simulink model "R2023b_Sim_Knickarmroboter_AndreasPaul"  (R2023b)
settings: Solver=ode45  StartTime=0.0  StopTime=2  MaxStep=3e-3  RelTol=1e-4  AbsTol=1e-7
values from neighbouring files (symbols this model uses):
  D = [1,0 ... (first row only)    [Initialisierung_Kickarmroboter.m]
  F_s1 = 8.5e-4    (= 0.00085)    [Initialisierung_Kickarmroboter.m]
  F_s2 = 3.2e-4    (= 0.00032)    [Initialisierung_Kickarmroboter.m]
  g = 9.81    [Initialisierung_Kickarmroboter.m]
  I = [1,0 ... (first row only)    [Initialisierung_Kickarmroboter.m]
  I1 = 0.0309    [Initialisierung_Kickarmroboter.m]
  I2 = 0.0045    [Initialisierung_Kickarmroboter.m]
  l1 = 0.16    [Initialisierung_Kickarmroboter.m]
  l2 = 0.128    [Initialisierung_Kickarmroboter.m]
  m1 = 0.1817    [Initialisierung_Kickarmroboter.m]
  m2 = 0.0944    [Initialisierung_Kickarmroboter.m]
  mu_v1 = 3.843e-6    (= 3.843e-06)    [Initialisierung_Kickarmroboter.m]
  mu_v2 = 3.887e-6    (= 3.887e-06)    [Initialisierung_Kickarmroboter.m]
  P = [1,0 ... (first row only)    [Initialisierung_Kickarmroboter.m]
  tau_delta_alpha = 0.1    [Initialisierung_Kickarmroboter.m]
  tau_delta_beta = 0.1    [Initialisierung_Kickarmroboter.m]
  x0 = [-2.5658; 0.2465; 0; 0]    [Initialisierung_Kickarmroboter.m]
libraries: simulink x1
settings Model: Creator=apaul  LastModifiedBy=apaul
settings RTWCC: GPUComputeCapability=5.0

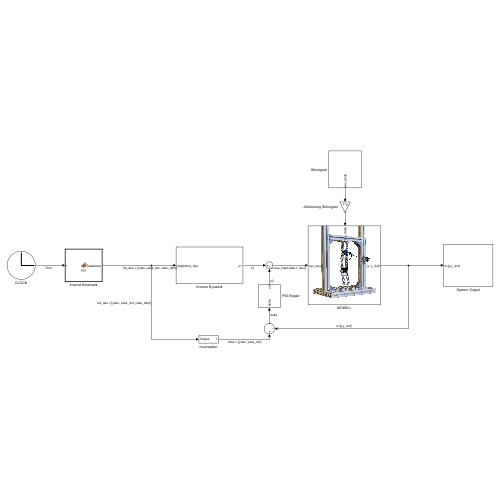
[thumbnail: Simulink's stored preview of the top-level diagram]
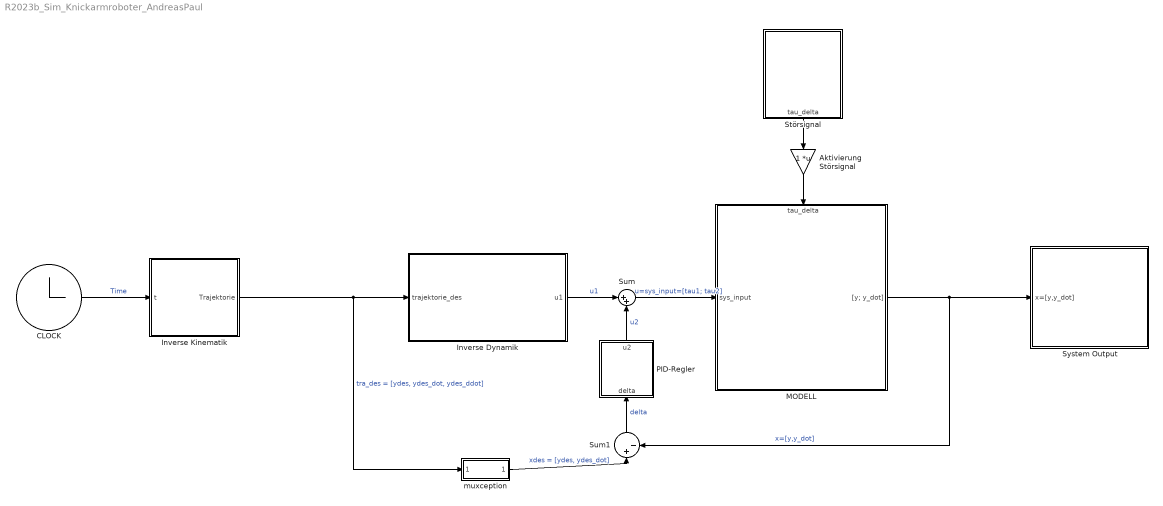
== system R2023b_Sim_Knickarmroboter_AndreasPaul ==
  Aktivierung Störsignal : Gain  Multiplication=Matrix(K*u)
  CLOCK : Clock
  Inverse Dynamik : Subsystem
  Inverse Kinematik : MATLAB Function  TreatAsAtomicUnit=on
  MODELL : Subsystem
      settings: PortSchema="{\"entries\":[{\"content\":{\"sides\":[{\"content\":{\"connectorIds\":[\"In1\"]},\"type\":\"ConnectorPlacement.EquallySpacedRectSide\",\"uuid\":\"e44e4c36-5739-4e55-a6ec-ca88d6f73c34\"},{\"content\":{\"connectorIds\":[\"Out1\"],\"side\":\"RIGHT\"},\"type\":\"ConnectorPlacement.EquallySpacedRectSide\",\"uuid\":\"5e6c41ef-5797-46fa-899e-46ee2542736a\"},{\"content\":{\"connectorIds\":[\"In2\"],\"side\":\"TOP\"},\"type\":\"ConnectorPlacement.EquallySpacedRectSide\",\"uuid\":\"f6ef0a2a-5723-4456-9106-f5bf4cdb5031\"}]},\"type\":\"ConnectorPlacement.EquallySpacedConnector\",\"uuid\":\"21cb76c5-3abe-4316-bc4d-4651aaedd4ba\"}],\"packageUris\":[\"http://schema.mathworks.com/mf0/Connector/R2020b\"],\"version\":\"1.0\"}"
      mask Display: image('Versuchsaufbau.png');
  PID-Regler : Subsystem
  Störsignal : Subsystem
  Sum : Sum  Inputs=|++
  Sum1 : Sum  Inputs=|+-
  System Output : Subsystem
  muxception : Subsystem
  wires:
  Sum/1 -> MODELL/1(sys_input)  "u=sys_input=[tau1; tau2]"
  Sum1/1 -> PID-Regler/1(delta)  "delta"
  MODELL/1("[y; y_dot]") -> System Output/1(x=[y,y_dot]), Sum1/2  "x=[y,y_dot]"
  Inverse Kinematik/1(Trajektorie) -> muxception/1(Output), Inverse Dynamik/1(trajektorie_des)  "tra_des = [ydes, ydes_dot, ydes_ddot]"
  Inverse Dynamik/1(u1) -> Sum/1  "u1"
  muxception/1(Out1) -> Sum1/1  "xdes = [ydes, ydes_dot]"
  CLOCK/1 -> Inverse Kinematik/1(t)  "Time"
  Störsignal/1(tau_delta) -> Aktivierung Störsignal/1
  Aktivierung Störsignal/1 -> MODELL/2(tau_delta)
  PID-Regler/1(u2) -> Sum/2  "u2"

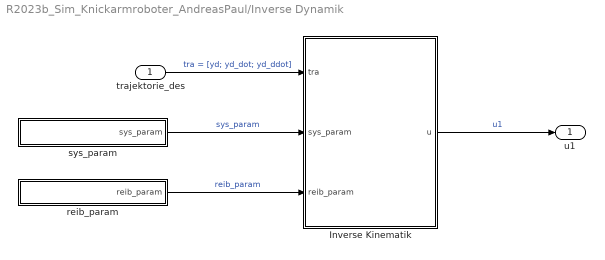
== system R2023b_Sim_Knickarmroboter_AndreasPaul/Inverse Dynamik ==
  trajektorie_des : Inport
  Inverse Kinematik : MATLAB Function  TreatAsAtomicUnit=on
  reib_param : Subsystem
  sys_param : Subsystem
  u1 : Outport
  wires:
  trajektorie_des/1 -> Inverse Kinematik/1(tra)  "tra = [yd; yd_dot; yd_ddot]"
  Inverse Kinematik/1(u) -> u1/1  "u1"
  sys_param/1(sys_param) -> Inverse Kinematik/2(sys_param)  "sys_param"
  reib_param/1(reib_param) -> Inverse Kinematik/3(reib_param)  "reib_param"

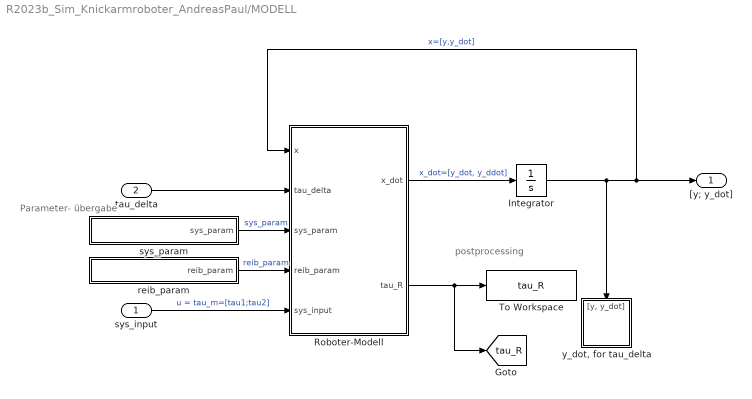
== system R2023b_Sim_Knickarmroboter_AndreasPaul/MODELL ==
  note: postprocessing
  note: Parameter-
      | übergabe
  sys_input : Inport
  tau_delta : Inport  Port=2
  Integrator : Integrator  InitialCondition=x0
  Roboter-Modell : MATLAB Function  TreatAsAtomicUnit=on
  To Workspace : ToWorkspace  VariableName=tau_R  SaveFormat=Timeseries  SampleTime=-1
  reib_param : Subsystem
  sys_param : Subsystem
  "y_dot, for tau_delta" : Subsystem
  "[y; y_dot]" : Outport
  tag scope: tau_R=global
  wires:
  Roboter-Modell/1(x_dot) -> Integrator/1  "x_dot=[y_dot, y_ddot]"
  Integrator/1 -> Roboter-Modell/1(x), "[y; y_dot]"/1, "y_dot, for tau_delta"/1("[y, y_dot]")  "x=[y,y_dot]"
  sys_input/1 -> Roboter-Modell/5(sys_input)  "u = tau_m=[tau1;tau2]"
  sys_param/1(sys_param) -> Roboter-Modell/3(sys_param)  "sys_param"
  reib_param/1(reib_param) -> Roboter-Modell/4(reib_param)  "reib_param"
  tau_delta/1 -> Roboter-Modell/2(tau_delta)
  Roboter-Modell/2(tau_R) -> [tau_R], To Workspace/1

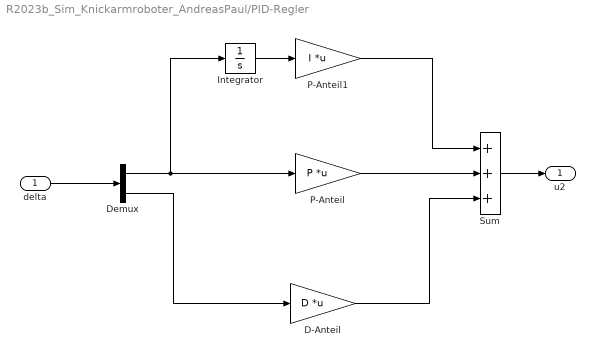
== system R2023b_Sim_Knickarmroboter_AndreasPaul/PID-Regler ==
  delta : Inport
  D-Anteil : Gain  Gain=D  Multiplication=Matrix(K*u)
  Demux : Demux  Outputs=2
  Integrator : Integrator
  P-Anteil : Gain  Gain=P  Multiplication=Matrix(K*u)
  P-Anteil1 : Gain  Gain=I  Multiplication=Matrix(K*u)
  Sum : Sum  Inputs=+++
  u2 : Outport
  wires:
  delta/1 -> Demux/1
  Demux/1 -> P-Anteil/1, Integrator/1
  Demux/2 -> D-Anteil/1
  Integrator/1 -> P-Anteil1/1
  Sum/1 -> u2/1
  P-Anteil1/1 -> Sum/1
  P-Anteil/1 -> Sum/2
  D-Anteil/1 -> Sum/3

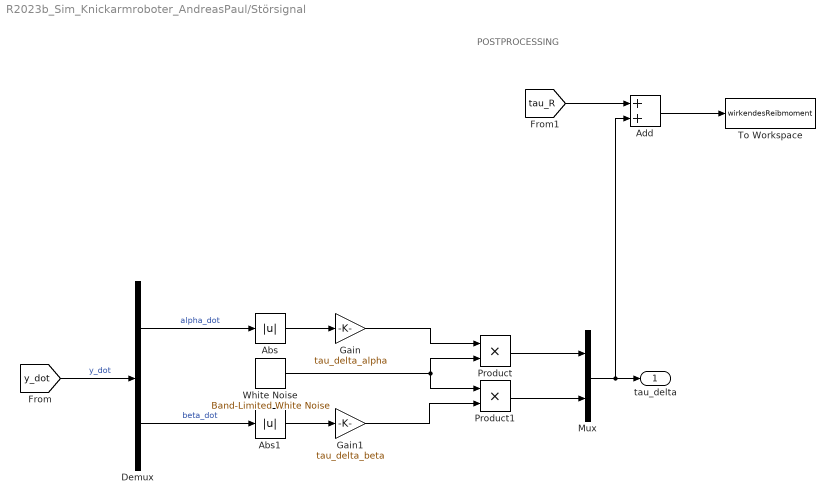
== system R2023b_Sim_Knickarmroboter_AndreasPaul/Störsignal ==
  note: POSTPROCESSING
  Abs : Abs  SaturateOnIntegerOverflow=off
  Abs1 : Abs  SaturateOnIntegerOverflow=off
  Add : Sum
  Demux : Demux  Outputs=2
  Gain : Gain  Gain=tau_delta_alpha
  Gain1 : Gain  Gain=tau_delta_beta
  Mux : Mux  Inputs=2
  Product : Product
  Product1 : Product
  To Workspace : ToWorkspace  VariableName=wirkendesReibmoment  SaveFormat=Timeseries  SampleTime=-1
  White Noise : simulink/Sources/Band-Limited White Noise  Cov=[0.1]  Ts=0.02  seed=[23341]
  tau_delta : Outport
  wires:
  [y_dot] -> Demux/1  "y_dot"
  Demux/1 -> Abs/1  "alpha_dot"
  Demux/2 -> Abs1/1  "beta_dot"
  Abs/1 -> Gain/1
  White Noise/1 -> Product1/1, Product/2
  Abs1/1 -> Gain1/1
  Product1/1 -> Mux/2
  Product/1 -> Mux/1
  Mux/1 -> tau_delta/1, Add/2
  Gain/1 -> Product/1
  Gain1/1 -> Product1/2
  [tau_R] -> Add/1
  Add/1 -> To Workspace/1

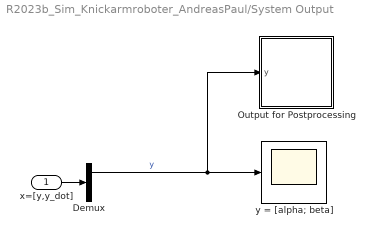
== system R2023b_Sim_Knickarmroboter_AndreasPaul/System Output ==
  x=[y,y_dot] : Inport
  Demux : Demux  Outputs=2
  Output for Postprocessing : Subsystem
  y = [alpha; beta] : Scope
  wires:
  Demux/1 -> Output for Postprocessing/1(y), y = [alpha; beta]/1  "y"
  x=[y,y_dot]/1 -> Demux/1

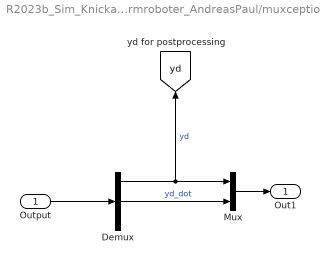
== system R2023b_Sim_Knickarmroboter_AndreasPaul/muxception ==
  Output : Inport
  Demux : Demux  Outputs=3
  Mux : Mux  Inputs=2
  Out1 : Outport
  tag scope: yd=global
  wires:
  Output/1 -> Demux/1
  Demux/1 -> Mux/1, [yd]  "yd"
  Demux/2 -> Mux/2  "yd_dot"
  Mux/1 -> Out1/1

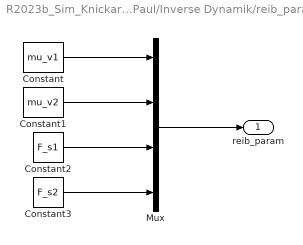
== system R2023b_Sim_Knickarmroboter_AndreasPaul/Inverse Dynamik/reib_param ==
  Constant : Constant  Value=mu_v1
  Constant1 : Constant  Value=mu_v2
  Constant2 : Constant  Value=F_s1
  Constant3 : Constant  Value=F_s2
  Mux : Mux
  reib_param : Outport
  wires:
  Constant3/1 -> Mux/4
  Constant2/1 -> Mux/3
  Constant1/1 -> Mux/2
  Constant/1 -> Mux/1
  Mux/1 -> reib_param/1

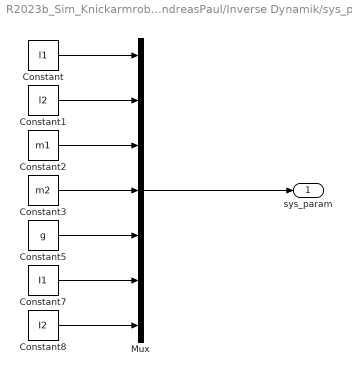
== system R2023b_Sim_Knickarmroboter_AndreasPaul/Inverse Dynamik/sys_param ==
  Constant : Constant  Value=l1
  Constant1 : Constant  Value=l2
  Constant2 : Constant  Value=m1
  Constant3 : Constant  Value=m2
  Constant5 : Constant  Value=g
  Constant7 : Constant  Value=I1
  Constant8 : Constant  Value=I2
  Mux : Mux  Inputs=7
  sys_param : Outport
  wires:
  Constant8/1 -> Mux/7
  Constant7/1 -> Mux/6
  Constant3/1 -> Mux/4
  Constant2/1 -> Mux/3
  Constant1/1 -> Mux/2
  Constant/1 -> Mux/1
  Mux/1 -> sys_param/1
  Constant5/1 -> Mux/5

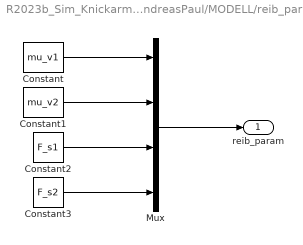
== system R2023b_Sim_Knickarmroboter_AndreasPaul/MODELL/reib_param ==
  Constant : Constant  Value=mu_v1
  Constant1 : Constant  Value=mu_v2
  Constant2 : Constant  Value=F_s1
  Constant3 : Constant  Value=F_s2
  Mux : Mux
  reib_param : Outport
  wires:
  Constant3/1 -> Mux/4
  Constant2/1 -> Mux/3
  Constant1/1 -> Mux/2
  Constant/1 -> Mux/1
  Mux/1 -> reib_param/1

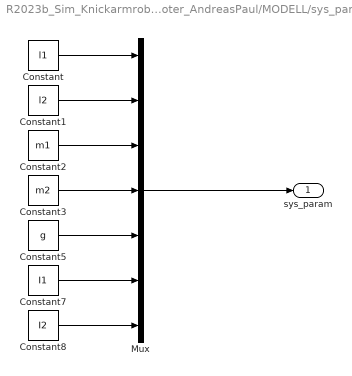
== system R2023b_Sim_Knickarmroboter_AndreasPaul/MODELL/sys_param ==
  Constant : Constant  Value=l1
  Constant1 : Constant  Value=l2
  Constant2 : Constant  Value=m1
  Constant3 : Constant  Value=m2
  Constant5 : Constant  Value=g
  Constant7 : Constant  Value=I1
  Constant8 : Constant  Value=I2
  Mux : Mux  Inputs=7
  sys_param : Outport
  wires:
  Constant8/1 -> Mux/7
  Constant7/1 -> Mux/6
  Constant3/1 -> Mux/4
  Constant2/1 -> Mux/3
  Constant1/1 -> Mux/2
  Constant/1 -> Mux/1
  Mux/1 -> sys_param/1
  Constant5/1 -> Mux/5

== system R2023b_Sim_Knickarmroboter_AndreasPaul/MODELL/y_dot, for tau_delta ==
  "[y, y_dot]" : Inport
  Demux : Demux  Outputs=2
  tag scope: y_dot=global
  wires:
  "[y, y_dot]"/1 -> Demux/1
  Demux/2 -> [y_dot]

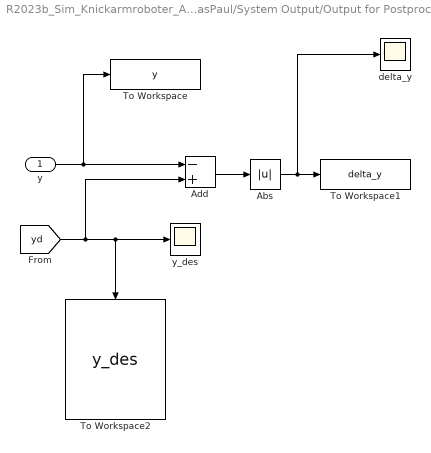
== system R2023b_Sim_Knickarmroboter_AndreasPaul/System Output/Output for Postprocessing ==
  y : Inport
  Abs : Abs  SaturateOnIntegerOverflow=off
  Add : Sum  Inputs=-+
  To Workspace : ToWorkspace  VariableName=y  SaveFormat=Timeseries  SampleTime=-1
  To Workspace1 : ToWorkspace  VariableName=delta_y  SaveFormat=Timeseries  SampleTime=-1
  To Workspace2 : ToWorkspace  VariableName=y_des  SaveFormat=Timeseries  SampleTime=-1
  delta_y : Scope
  y_des : Scope
  wires:
  y/1 -> Add/1, To Workspace/1
  [yd] -> To Workspace2/1, y_des/1, Add/2
  Add/1 -> Abs/1
  Abs/1 -> delta_y/1, To Workspace1/1

== matlab function R2023b_Sim_Knickarmroboter_AndreasPaul/Inverse Dynamik/Inverse Kinematik ==
  data: tra input; u output; sys_param input; reib_param input
function u = fcn(tra, sys_param, reib_param)

M = calc_M(tra(1:2), sys_param);
D = calc_D(tra(1:2), tra(3:4), sys_param);
G = calc_G(tra(1:2), sys_param);
tau_R = calc_tau_R(tra(1:2), tra(3:4), sys_param, reib_param);
B = eye(2,2);

u = B \ (M * tra(5:6) + D * tra(3:4) + G - tau_R);
end

== matlab function R2023b_Sim_Knickarmroboter_AndreasPaul/MODELL/Roboter-Modell ==
  data: x input; tau_delta input; sys_param input; reib_param input; x_dot output; sys_input input; tau_R output
function [x_dot, tau_R] = fcn(x, tau_delta, sys_param, reib_param, sys_input)
%x(1:2)=y
%x(3:4)=y_dot
M = calc_M(x(1:2), sys_param);
D = calc_D(x(1:2), x(3:4), sys_param);
G = calc_G(x(1:2), sys_param);
tau_R = calc_tau_R(x(1:2), x(3:4), sys_param, reib_param);

%State Space System
x_dot = [x(3:4);
         M \ ((tau_R + tau_delta) + sys_input - G - D * x(3:4))];

% %Singularität sobald ich D und sys_input in die Inversion einbeziehe
% x_dot = [x(3:4);
%          M \ ((tau_R + tau_delta) - G) - D * x(3:4) + sys_input];
end

== matlab function R2023b_Sim_Knickarmroboter_AndreasPaul/Inverse Kinematik ==
  data: t input; Trajektorie output
function Trajektorie = fcn(t)

tra = calc_Trajektorie_verallg(t);

Trajektorie = tra;
